simulink model "exp_3"  (R2013b)
settings: Solver=ode3  StartTime=0.0  StopTime=10.0  FixedStep=0.02  RelTol=1e-3
libraries: simulink x1
settings Model: Creator=lenovo  LastModifiedBy=lenovo

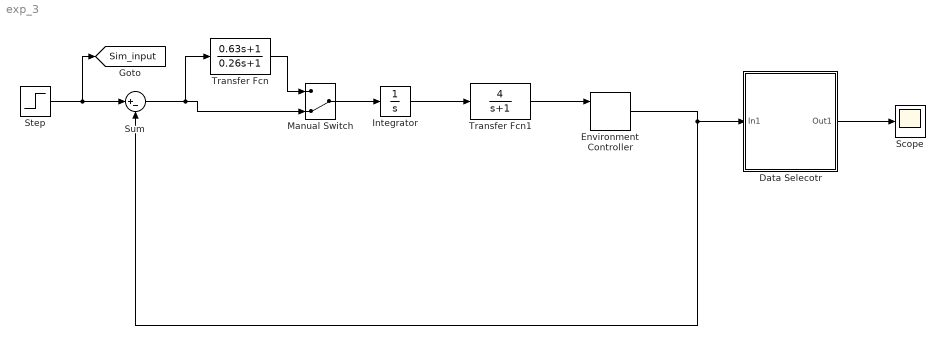
== system exp_3 ==
  Data Selecotr : Subsystem
      mask Display:
      | port_label('input',1,'output')
      | port_label('output',1,'scope')
  Environment Controller : simulink/Signal Routing/Environment Controller
  Integrator : Integrator
  Manual Switch : ManualSwitch  CurrentSetting=0
  Scope : Scope
  Step : Step  SampleTime=0
  Sum : Sum  Inputs=|+-
  Transfer Fcn : TransferFcn  Numerator=[0.63 1]  Denominator=[0.26 1]
  Transfer Fcn1 : TransferFcn  Numerator=[4]  Denominator=[1 1]
  tag scope: Sim_input=global
  wires:
  Step/1 -> [Sim_input], Sum/1
  Sum/1 -> Transfer Fcn/1, Manual Switch/2
  Transfer Fcn/1 -> Manual Switch/1
  Manual Switch/1 -> Integrator/1
  Integrator/1 -> Transfer Fcn1/1
  Transfer Fcn1/1 -> Environment Controller/1
  Environment Controller/1 -> Sum/2, Data Selecotr/1(In1)
  Data Selecotr/1(Out1) -> Scope/1

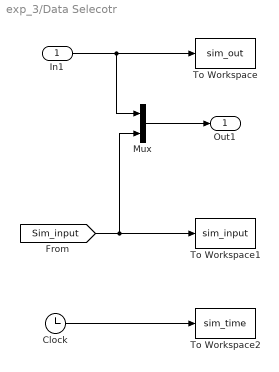
== system exp_3/Data Selecotr ==
  In1 : Inport
  Clock : Clock
  Mux : Mux  Inputs=2
  To Workspace : ToWorkspace  VariableName=sim_out  SampleTime=-1  SaveFormat=Timeseries
  To Workspace1 : ToWorkspace  VariableName=sim_input  SampleTime=-1  SaveFormat=Timeseries
  To Workspace2 : ToWorkspace  VariableName=sim_time  SampleTime=-1  SaveFormat=Timeseries
  Out1 : Outport
  wires:
  In1/1 -> Mux/1, To Workspace/1
  Mux/1 -> Out1/1
  Clock/1 -> To Workspace2/1
  [Sim_input] -> To Workspace1/1, Mux/2
